simulink model "AMCLIB_BemfObsrvDQ_BAM"  (Simulink 9.3)
settings: Solver=VariableStepAuto  StartTime=0.0  StopTime=10.0  RelTol=1e-3
settings Model: Creator=nxa18952  LastModifiedBy=nxa18952
settings DataIOCC: SaveFormat=Dataset  SignalLoggingSaveFormat=Dataset  ReturnWorkspaceOutputs=on
settings OptimizationCC: LifeSpan=auto
settings DebuggingCC: UnderspecifiedInitializationDetection=Simplified  MergeDetectMultiDrivingBlocksExec=error  FcnCallInpInsideContextMsg=error  SFUnexpectedBacktrackingDiag=error  SFNoUnconditionalDefaultTransitionDiag=error  SFExecutionAtInitializationDiag=warning  ArithmeticOperatorsInVariantConditions=error
settings HardwareCC: ProdBitPerPointer=64  ProdBitPerSizeT=64  ProdBitPerPtrDiffT=64  ProdLargestAtomicFloat=Float  ProdIntDivRoundTo=Zero  ProdEndianess=LittleEndian  ProdWordSize=64  ProdHWDeviceType=Intel->x86-64 (Windows64)
settings ModelReferenceCC: PropagateSignalLabelsOutOfModel=on
settings SFSimCC: SimUseLocalCustomCode=on
settings RTWCC: RTWUseLocalCustomCode=on
settings CodeAppCC: StateflowObjectComments=off
settings GRTTargetCC: TargetLangStandard=C99 (ISO)  CombineOutputUpdateFcns=on  GRTInterface=off
settings ConfigComp: CovMetricSettings=dwe  CovHtmlReporting=off  CovSaveCumulativeToWorkspaceVar=off  CovSaveSingleToWorkspaceVar=off  CovExternalEMLEnable=on

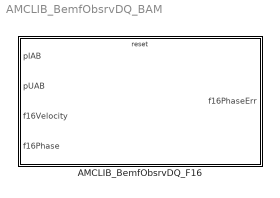
== system AMCLIB_BemfObsrvDQ_BAM ==
  AMCLIB_BemfObsrvDQ_F16 : Subsystem  TreatAsAtomicUnit=on  mask(AMCLIB_BemfObsrvDQ_F16){showStates=Hide (faster execution), resetStatesEnable=Pre-set according to the first set of inputs after reset, f16IGain=0, f16UGain=0, f16WIGain=0, f16EGain=0, s16Shift=0, f16CC1sc_D=0, f16CC2sc_D=0, f16UpperLimit_D=0, f16LowerLimit_D=0, f16CC1sc_Q=0, f16CC2sc_Q=0, f16UpperLimit_Q=0, f16LowerLimit_Q=0, u16NShift=0}
      mask prompts: showStates "Show internal states"; resetStatesEnable "Internal state after reset"; f16IGain "f16IGain (Scaled RL circuit constant)"; f16UGain "f16UGain (Scaled voltage cross-coupling constant)"; f16WIGain "f16WIGain (Scaled angular velocity cross-coupling constant)"; f16EGain "f16EGain (Scaled back-EMF cross-coupling constant)"; s16Shift "s16Shift (Scaling bitwise shift applied to all cross-coupling constants)"; f16CC1sc_D "f16CC1sc_D (CC1 coefficient of the D-axis PI controller)"; f16CC2sc_D "f16CC2sc_D (CC2 coefficient of the D-axis PI controller)"; f16UpperLimit_D "f16UpperLimit_D (Upper Limit of the D-axis PI controller)"; f16LowerLimit_D "f16LowerLimit_D (Lower Limit of the D-axis PI controller)"; f16CC1sc_Q "f16CC1sc_Q (CC1 coefficient of the Q-axis PI controller)"; f16CC2sc_Q "f16CC2sc_Q (CC2 coefficient of the Q-axis PI controller)"; f16UpperLimit_Q "f16UpperLimit_Q (Upper Limit of the Q-axis PI controller)"; f16LowerLimit_Q "f16LowerLimit_Q (Lower Limit of the Q-axis PI controller)"; u16NShift "u16NShift (Scaling bitwise shift applied to the controller coefficients)"
      mask help: PMSM back-EMF observer DQ in 16-bit fixed-point fractional implementation. This block supports re-initialization of the internal state during simulation. If the block is reset, the observer will align with the motor's position and speed measured in the next time step. This allows seamless on-the-fly transition to the closed-loop control. Refer to the AMMCLIB User's Guide for further details.
      mask init:
      | if ~evalin('base','exist(''tS8'',''var'')')
      |   if (2 ~= exist('SWLIBS_Typedefs.mat','file'))
      |       error('File SWLIBS_Typedefs.mat is not on the Matlab path. Please add the AMMCLIB "bam" folder in the Matlab Search Path.');
      |   else
      |       evalin('base', 'load(''SWLIBS_Typedefs.mat'')');
      |   end
      | end
      | if showStates == 1
      |     % hidden state variables
      |     if strcmp(get_param([gcb '/f16IGain'], 'BlockType'), 'Inport')
      |         posblk = get_param(gcb, 'Position');
      | 
      |         pos = get_param(    [gcb, '/f16IGain'], 'Position');
      |         orient = get_param( [gcb, '/f16IGain'], 'Orientation');
      |         delete_block(       [gcb, '/f16IGain']);
      |         add_block('built-in/Ground', [gcb, '/f16IGain'], 'Position', pos, 'Orientation', orient);
      | 
      |         pos = get_param(    [gcb, '/f16UGain'], 'Position');
      |         orient = get_param( [gcb, '/f16UGain'], 'Orientation');
      |         delete_block(       [gcb, '/f16UGain']);
      |         add_block('built-in/Ground', [gcb, '/f16UGain'], 'Position', pos, 'Orientation', orient);
      | 
      |         pos = get_param(    [gcb, '/f16WIGain'], 'Position');
      |         orient = get_param( [gcb, '/f16WIGain'], 'Orientation');
      |         delete_block(       [gcb, '/f16WIGain']);
      |         add_block('built-in/Ground', [gcb, '/f16WIGain'], 'Position', pos, 'Orientation', orient);
      | 
      |         pos = get_param(    [gcb, '/f16EGain'], 'Position');
      |         orient = get_param( [gcb, '/f16EGain'], 'Orientation');
      |         delete_block(       [gcb, '/f16EGain']);
      |         add_block('built-in/Ground', [gcb, '/f16EGain'], 'Position', pos, 'Orientation', orient);
      | 
      |         pos = get_param(    [gcb, '/s16Shift'], 'Position');
      |         orient = get_param( [gcb, '/s16Shift'], 'Orientation');
      |         delete_block(       [gcb, '/s16Shift']);
      |         add_block('built-in/Ground', [gcb, '/s16Shift'], 'Position', pos, 'Orientation', orient);
      | 
      |         pos = get_param(    [gcb, '/f16CC1sc_D'], 'Position');
      |         orient = get_param( [gcb, '/f16CC1sc_D'], 'Orientation');
      |         delete_block(       [gcb, '/f16CC1sc_D']);
      |         add_block('built-in/Ground', [gcb, '/f16CC1sc_D'], 'Position', pos, 'Orientation', orient);
      | 
      |         pos = get_param(    [gcb, '/f16CC2sc_D'], 'Position');
      |         orient = get_param( [gcb, '/f16CC2sc_D'], 'Orientation');
      |         delete_block(       [gcb, '/f16CC2sc_D']);
      |         add_block('built-in/Ground', [gcb, '/f16CC2sc_D'], 'Position', pos, 'Orientation', orient);
      | 
      |         pos = get_param(    [gcb, '/f16UpperLimit_D'], 'Position');
      |         orient = get_param( [gcb, '/f16UpperLimit_D'], 'Orientation');
      |         delete_block(       [gcb, '/f16UpperLimit_D']);
      |         add_block('built-in/Ground', [gcb, '/f16UpperLimit_D'], 'Position', pos, 'Orientation', orient);
      | 
      |         pos = get_param(    [gcb, '/f16LowerLimit_D'], 'Position');
      |         orient = get_param( [gcb, '/f16LowerLimit_D'], 'Orientation');
      |         delete_block(       [gcb, '/f16LowerLimit_D']);
      |         add_block('built-in/Ground', [gcb, '/f16LowerLimit_D'], 'Position', pos, 'Orientation', orient);
      | 
      |         pos = get_param(    [gcb, '/f16CC1sc_Q'], 'Position');
      |         orient = get_param( [gcb, '/f16CC1sc_Q'], 'Orientation');
      |         delete_block(       [gcb, '/f16CC1sc_Q']);
      |         add_block('built-in/Ground', [gcb, '/f16CC1sc_Q'], 'Position', pos, 'Orientation', orient);
      | 
      |         pos = get_param(    [gcb, '/f16CC2sc_Q'], 'Position');
      |         orient = get_param( [gcb, '/f16CC2sc_Q'], 'Orientation');
      |         delete_block(       [gcb, '/f16CC2sc_Q']);
      |         add_block('built-in/Ground', [gcb, '/f16CC2sc_Q'], 'Position', pos, 'Orientation', orient);
      | 
      |         pos = get_param(    [gcb, '/f16UpperLimit_Q'], 'Position');
      |         orient = get_param( [gcb, '/f16UpperLimit_Q'], 'Orientation');
      |         delete_block(       [gcb, '/f16UpperLimit_Q']);
      |         add_block('built-in/Ground', [gcb, '/f16UpperLimit_Q'], 'Position', pos, 'Orientation', orient);
      | 
      |         pos = get_param(    [gcb, '/f16LowerLimit_Q'], 'Position');
      |         orient = get_param( [gcb, '/f16LowerLimit_Q'], 'Orientation');
      |         delete_block(       [gcb, '/f16LowerLimit_Q']);
      |         add_block('built-in/Ground', [gcb, '/f16LowerLimit_Q'], 'Position', pos, 'Orientation', orient);
      | 
      |         pos = get_param(    [gcb, '/u16NShift'], 'Position');
      |         orient = get_param( [gcb, '/u16NShift'], 'Orientation');
      |         delete_block(       [gcb, '/u16NShift']);
      |         add_block('built-in/Ground', [gcb, '/u16NShift'], 'Position', pos, 'Orientation', orient);
      | 
      |         pos = get_param(    [gcb, '/f32Acc_D'], 'Position');
      |         orient = get_param( [gcb, '/f32Acc_D'], 'Orientation');
      |         delete_block(       [gcb, '/f32Acc_D']);
      |         add_block('built-in/Ground', [gcb, '/f32Acc_D'], 'Position', pos, 'Orientation', orient);
      | 
      |         pos = get_param(    [gcb, '/f16InErrK1_D'], 'Position');
      |         orient = get_param( [gcb, '/f16InErrK1_D'], 'Orientation');
      |         delete_block(       [gcb, '/f16InErrK1_D']);
      |         add_block('built-in/Ground', [gcb, '/f16InErrK1_D'], 'Position', pos, 'Orientation', orient);
      | 
      |         pos = get_param(    [gcb, '/f32Acc_Q'], 'Position');
      |         orient = get_param( [gcb, '/f32Acc_Q'], 'Orientation');
      |         delete_block(       [gcb, '/f32Acc_Q']);
      |         add_block('built-in/Ground', [gcb, '/f32Acc_Q'], 'Position', pos, 'Orientation', orient);
      | 
      |         pos = get_param(    [gcb, '/f16InErrK1_Q'], 'Position');
      |         orient = get_param( [gcb, '/f16InErrK1_Q'], 'Orientation');
      |         delete_block(       [gcb, '/f16InErrK1_Q']);
      |         add_block('built-in/Ground', [gcb, '/f16InErrK1_Q'], 'Position', pos, 'Orientation', orient);
      | 
      |         pos = get_param(    [gcb, '/f32IObsrvIn_1L_D'], 'Position');
      |         orient = get_param( [gcb, '/f32IObsrvIn_1L_D'], 'Orientation');
      |         delete_block(       [gcb, '/f32IObsrvIn_1L_D']);
      |         add_block('built-in/Ground', [gcb, '/f32IObsrvIn_1L_D'], 'Position', pos, 'Orientation', orient);
      | 
      |         pos = get_param(    [gcb, '/f16IObsrvIn_1H_D'], 'Position');
      |         orient = get_param( [gcb, '/f16IObsrvIn_1H_D'], 'Orientation');
      |         delete_block(       [gcb, '/f16IObsrvIn_1H_D']);
      |         add_block('built-in/Ground', [gcb, '/f16IObsrvIn_1H_D'], 'Position', pos, 'Orientation', orient);
      | 
      |         pos = get_param(    [gcb, '/f32IObsrvIn_1L_Q'], 'Position');
      |         orient = get_param( [gcb, '/f32IObsrvIn_1L_Q'], 'Orientation');
      |         delete_block(       [gcb, '/f32IObsrvIn_1L_Q']);
      |         add_block('built-in/Ground', [gcb, '/f32IObsrvIn_1L_Q'], 'Position', pos, 'Orientation', orient);
      | 
      |         pos = get_param(    [gcb, '/f16IObsrvIn_1H_Q'], 'Position');
      |         orient = get_param( [gcb, '/f16IObsrvIn_1H_Q'], 'Orientation');
      |         delete_block(       [gcb, '/f16IObsrvIn_1H_Q']);
      |         add_block('built-in/Ground', [gcb, '/f16IObsrvIn_1H_Q'], 'Position', pos, 'Orientation', orient);
      | 
      |         pos = get_param(    [gcb, '/f32IObsrv_D'], 'Position');
      |         orient = get_param( [gcb, '/f32IObsrv_D'], 'Orientation');
      |         delete_block(       [gcb, '/f32IObsrv_D']);
      |         add_block('built-in/Ground', [gcb, '/f32IObsrv_D'], 'Position', pos, 'Orientation', orient);
      | 
      |         pos = get_param(    [gcb, '/f32IObsrv_Q'], 'Position');
      |         orient = get_param( [gcb, '/f32IObsrv_Q'], 'Orientation');
      |         delete_block(       [gcb, '/f32IObsrv_Q']);
      |         add_block('built-in/Ground', [gcb, '/f32IObsrv_Q'], 'Position', pos, 'Orientation', orient);
      | 
      | 
      |         pos = get_param(    [gcb '/f16EObsrv_D_Out'], 'Position');
      |         orient = get_param( [gcb '/f16EObsrv_D_Out'], 'Orientation');
      |         delete_block(       [gcb '/f16EObsrv_D_Out']);
      |         add_block('built-in/Terminator', [gcb '/f16EObsrv_D_Out'], 'Position', pos, 'Orientation', orient);
      | 
      |         pos = get_param(    [gcb '/f16EObsrv_Q_Out'], 'Position');
      |         orient = get_param( [gcb '/f16EObsrv_Q_Out'], 'Orientation');
      |         delete_block(       [gcb '/f16EObsrv_Q_Out']);
      |         add_block('built-in/Terminator', [gcb '/f16EObsrv_Q_Out'], 'Position', pos, 'Orientation', orient);
      | 
      |         pos = get_param(    [gcb '/f32Acc_D_Out'], 'Position');
      |         orient = get_param( [gcb '/f32Acc_D_Out'], 'Orientation');
      |         delete_block(       [gcb '/f32Acc_D_Out']);
      |         add_block('built-in/Terminator', [gcb '/f32Acc_D_Out'], 'Position', pos, 'Orientation', orient);
      | 
      |         pos = get_param(    [gcb '/f16InErrK1_D_Out'], 'Position');
      |         orient = get_param( [gcb '/f16InErrK1_D_Out'], 'Orientation');
      |         delete_block(       [gcb '/f16InErrK1_D_Out']);
      |         add_block('built-in/Terminator', [gcb '/f16InErrK1_D_Out'], 'Position', pos, 'Orientation', orient);
      | 
      |         pos = get_param(    [gcb '/f32Acc_Q_Out'], 'Position');
      |         orient = get_param( [gcb '/f32Acc_Q_Out'], 'Orientation');
      |         delete_block(       [gcb '/f32Acc_Q_Out']);
      |         add_block('built-in/Terminator', [gcb '/f32Acc_Q_Out'], 'Position', pos, 'Orientation', orient);
      | 
      |         pos = get_param(    [gcb '/f16InErrK1_Q_Out'], 'Position');
      |         orient = get_param( [gcb '/f16InErrK1_Q_Out'], 'Orientation');
      |         delete_block(       [gcb '/f16InErrK1_Q_Out']);
      |         add_block('built-in/Terminator', [gcb '/f16InErrK1_Q_Out'], 'Position', pos, 'Orientation', orient);
      | 
      |         pos = get_param(    [gcb '/f32IObsrvIn_1L_D_Out'], 'Position');
      |         orient = get_param( [gcb '/f32IObsrvIn_1L_D_Out'], 'Orientation');
      |         delete_block(       [gcb '/f32IObsrvIn_1L_D_Out']);
      |         add_block('built-in/Terminator', [gcb '/f32IObsrvIn_1L_D_Out'], 'Position', pos, 'Orientation', orient);
      | 
      |         pos = get_param(    [gcb '/f16IObsrvIn_1H_D_Out'], 'Position');
      |         orient = get_param( [gcb '/f16IObsrvIn_1H_D_Out'], 'Orientation');
      |         delete_block(       [gcb '/f16IObsrvIn_1H_D_Out']);
      |         add_block('built-in/Terminator', [gcb '/f16IObsrvIn_1H_D_Out'], 'Position', pos, 'Orientation', orient);
      | 
      |         pos = get_param(    [gcb '/f32IObsrvIn_1L_Q_Out'], 'Position');
      |         orient = get_param( [gcb '/f32IObsrvIn_1L_Q_Out'], 'Orientation');
      |         delete_block(       [gcb '/f32IObsrvIn_1L_Q_Out']);
      |         add_block('built-in/Terminator', [gcb '/f32IObsrvIn_1L_Q_Out'], 'Position', pos, 'Orientation', orient);
      | 
      |         pos = get_param(    [gcb '/f16IObsrvIn_1H_Q_Out'], 'Position');
      |         orient = get_param( [gcb '/f16IObsrvIn_1H_Q_Out'], 'Orientation');
      |         delete_block(       [gcb '/f16IObsrvIn_1H_Q_Out']);
      |         add_block('built-in/Terminator', [gcb '/f16IObsrvIn_1H_Q_Out'], 'Position', pos, 'Orientation', orient);
      | 
      |         pos = get_param(    [gcb '/f32IObsrv_D_Out'], 'Position');
      |         orient = get_param( [gcb '/f32IObsrv_D_Out'], 'Orientation');
      |         delete_block(       [gcb '/f32IObsrv_D_Out']);
      |         add_block('built-in/Terminator', [gcb '/f32IObsrv_D_Out'], 'Position', pos, 'Orientation', orient);
      | 
      |         pos = get_param(    [gcb '/f32IObsrv_Q_Out'], 'Position');
      |         orient = get_param( [gcb '/f32IObsrv_Q_Out'], 'Orientation');
      |         delete_block(       [gcb '/f32IObsrv_Q_Out']);
      |         add_block('built-in/Terminator', [gcb '/f32IObsrv_Q_Out'], 'Position', pos, 'Orientation', orient);
      | 
      | 
      |         set_param([gcb '/pIAB'], 'Port', '1');
      |         set_param([gcb '/pUAB'], 'Port', '2');
      |         set_param([gcb '/f16Velocity'], 'Port', '3');
      |         set_param([gcb '/f16Phase'], 'Port', '4');
      | 
      |         set_param([gcb '/f16PhaseErr'], 'Port', '1');
      | 
      |         set_param(gcb,'MaskEnables',{'on','on','on','on','on','on','on','on','on','on','on','on','on','on','on','on'});
      | 
      |         if (posblk(4) - posblk(2)) > 125
      |           height = 125;
      |           set_param(gcb,'Position',[posblk(1), posblk(2), posblk(3), posblk(2)+height])
      |         end
      |     end
      | else
      |     % shown state variables
      |     if strcmp(get_param([gcb '/f16IGain'], 'BlockType'), 'Ground')
      |         posblk = get_param(gcb, 'Position');
      | 
      |         pos = get_param(    [gcb, '/f16IGain'], 'Position');
      |         orient = get_param( [gcb, '/f16IGain'], 'Orientation');
      |         delete_block(       [gcb, '/f16IGain']);
      |         add_block('built-in/Inport', [gcb, '/f16IGain'], 'Position', pos, 'Orientation', orient, 'OutDataTypeStr', 'int16');
      | 
      |         pos = get_param(    [gcb, '/f16UGain'], 'Position');
      |         orient = get_param( [gcb, '/f16UGain'], 'Orientation');
      |         delete_block(       [gcb, '/f16UGain']);
      |         add_block('built-in/Inport', [gcb, '/f16UGain'], 'Position', pos, 'Orientation', orient, 'OutDataTypeStr', 'int16');
      | 
      |         pos = get_param(    [gcb, '/f16WIGain'], 'Position');
      |         orient = get_param( [gcb, '/f16WIGain'], 'Orientation');
      |         delete_block(       [gcb, '/f16WIGain']);
      |         add_block('built-in/Inport', [gcb, '/f16WIGain'], 'Position', pos, 'Orientation', orient, 'OutDataTypeStr', 'int16');
      | 
      |         pos = get_param(    [gcb, '/f16EGain'], 'Position');
      |         orient = get_param( [gcb, '/f16EGain'], 'Orientation');
      |         delete_block(       [gcb, '/f16EGain']);
      |         add_block('built-in/Inport', [gcb, '/f16EGain'], 'Position', pos, 'Orientation', orient, 'OutDataTypeStr', 'int16');
      | 
      |         pos = get_param(    [gcb, '/s16Shift'], 'Position');
      |         orient = get_param( [gcb, '/s16Shift'], 'Orientation');
      |         delete_block(       [gcb, '/s16Shift']);
      |         add_block('built-in/Inport', [gcb, '/s16Shift'], 'Position', pos, 'Orientation', orient, 'OutDataTypeStr', 'int16');
      | 
      |         pos = get_param(    [gcb, '/f16CC1sc_D'], 'Position');
      |         orient = get_param( [gcb, '/f16CC1sc_D'], 'Orientation');
      |         delete_block(       [gcb, '/f16CC1sc_D']);
      |         add_block('built-in/Inport', [gcb, '/f16CC1sc_D'], 'Position', pos, 'Orientation', orient, 'OutDataTypeStr', 'int16');
      | 
      |         pos = get_param(    [gcb, '/f16CC2sc_D'], 'Position');
      |         orient = get_param( [gcb, '/f16CC2sc_D'], 'Orientation');
      |         delete_block(       [gcb, '/f16CC2sc_D']);
      |         add_block('built-in/Inport', [gcb, '/f16CC2sc_D'], 'Position', pos, 'Orientation', orient, 'OutDataTypeStr', 'int16');
      | 
      |         pos = get_param(    [gcb, '/f16UpperLimit_D'], 'Position');
      |         orient = get_param( [gcb, '/f16UpperLimit_D'], 'Orientation');
      |         delete_block(       [gcb, '/f16UpperLimit_D']);
      |         add_block('built-in/Inport', [gcb, '/f16UpperLimit_D'], 'Position', pos, 'Orientation', orient, 'OutDataTypeStr', 'int16');
      | 
      |         pos = get_param(    [gcb, '/f16LowerLimit_D'], 'Position');
      |         orient = get_param( [gcb, '/f16LowerLimit_D'], 'Orientation');
      |         delete_block(       [gcb, '/f16LowerLimit_D']);
      |         add_block('built-in/Inport', [gcb, '/f16LowerLimit_D'], 'Position', pos, 'Orientation', orient, 'OutDataTypeStr', 'int16');
      | 
      |         pos = get_param(    [gcb, '/f16CC1sc_Q'], 'Position');
      |         orient = get_param( [gcb, '/f16CC1sc_Q'], 'Orientation');
      |         delete_block(       [gcb, '/f16CC1sc_Q']);
      |         add_block('built-in/Inport', [gcb, '/f16CC1sc_Q'], 'Position', pos, 'Orientation', orient, 'OutDataTypeStr', 'int16');
      | 
      |         pos = get_param(    [gcb, '/f16CC2sc_Q'], 'Position');
      |         orient = get_param( [gcb, '/f16CC2sc_Q'], 'Orientation');
      |         delete_block(       [gcb, '/f16CC2sc_Q']);
      |         add_block('built-in/Inport', [gcb, '/f16CC2sc_Q'], 'Position', pos, 'Orientation', orient, 'OutDataTypeStr', 'int16');
      | 
      |         pos = get_param(    [gcb, '/f16UpperLimit_Q'], 'Position');
      |         orient = get_param( [gcb, '/f16UpperLimit_Q'], 'Orientation');
      |         delete_block(       [gcb, '/f16UpperLimit_Q']);
      |         add_block('built-in/Inport', [gcb, '/f16UpperLimit_Q'], 'Position', pos, 'Orientation', orient, 'OutDataTypeStr', 'int16');
      | 
      |         pos = get_param(    [gcb, '/f16LowerLimit_Q'], 'Position');
      |         orient = get_param( [gcb, '/f16LowerLimit_Q'], 'Orientation');
      |         delete_block(       [gcb, '/f16LowerLimit_Q']);
      |         add_block('built-in/Inport', [gcb, '/f16LowerLimit_Q'], 'Position', pos, 'Orientation', orient, 'OutDataTypeStr', 'int16');
      | 
      |         pos = get_param(    [gcb, '/u16NShift'], 'Position');
      |         orient = get_param( [gcb, '/u16NShift'], 'Orientation');
      |         delete_block(       [gcb, '/u16NShift']);
      |         add_block('built-in/Inport', [gcb, '/u16NShift'], 'Position', pos, 'Orientation', orient, 'OutDataTypeStr', 'uint16');
      | 
      |         pos = get_param(    [gcb, '/f32Acc_D'], 'Position');
      |         orient = get_param( [gcb, '/f32Acc_D'], 'Orientation');
      |         delete_block(       [gcb, '/f32Acc_D']);
      |         add_block('built-in/Inport', [gcb, '/f32Acc_D'], 'Position', pos, 'Orientation', orient, 'OutDataTypeStr', 'int32');
      | 
      |         pos = get_param(    [gcb, '/f16InErrK1_D'], 'Position');
      |         orient = get_param( [gcb, '/f16InErrK1_D'], 'Orientation');
      |         delete_block(       [gcb, '/f16InErrK1_D']);
      |         add_block('built-in/Inport', [gcb, '/f16InErrK1_D'], 'Position', pos, 'Orientation', orient, 'OutDataTypeStr', 'int16');
      | 
      |         pos = get_param(    [gcb, '/f32Acc_Q'], 'Position');
      |         orient = get_param( [gcb, '/f32Acc_Q'], 'Orientation');
      |         delete_block(       [gcb, '/f32Acc_Q']);
      |         add_block('built-in/Inport', [gcb, '/f32Acc_Q'], 'Position', pos, 'Orientation', orient, 'OutDataTypeStr', 'int32');
      | 
      |         pos = get_param(    [gcb, '/f16InErrK1_Q'], 'Position');
      |         orient = get_param( [gcb, '/f16InErrK1_Q'], 'Orientation');
      |         delete_block(       [gcb, '/f16InErrK1_Q']);
      |         add_block('built-in/Inport', [gcb, '/f16InErrK1_Q'], 'Position', pos, 'Orientation', orient, 'OutDataTypeStr', 'int16');
      | 
      |         pos = get_param(    [gcb, '/f32IObsrvIn_1L_D'], 'Position');
      |         orient = get_param( [gcb, '/f32IObsrvIn_1L_D'], 'Orientation');
      |         delete_block(       [gcb, '/f32IObsrvIn_1L_D']);
      |         add_block('built-in/Inport', [gcb, '/f32IObsrvIn_1L_D'], 'Position', pos, 'Orientation', orient, 'OutDataTypeStr', 'int32');
      | 
      |         pos = get_param(    [gcb, '/f16IObsrvIn_1H_D'], 'Position');
      |         orient = get_param( [gcb, '/f16IObsrvIn_1H_D'], 'Orientation');
      |         delete_block(       [gcb, '/f16IObsrvIn_1H_D']);
      |         add_block('built-in/Inport', [gcb, '/f16IObsrvIn_1H_D'], 'Position', pos, 'Orientation', orient, 'OutDataTypeStr', 'int16');
      | 
      |         pos = get_param(    [gcb, '/f32IObsrvIn_1L_Q'], 'Position');
      |         orient = get_param( [gcb, '/f32IObsrvIn_1L_Q'], 'Orientation');
      |         delete_block(       [gcb, '/f32IObsrvIn_1L_Q']);
      |         add_block('built-in/Inport', [gcb, '/f32IObsrvIn_1L_Q'], 'Position', pos, 'Orientation', orient, 'OutDataTypeStr', 'int32');
      | 
      |         pos = get_param(    [gcb, '/f16IObsrvIn_1H_Q'], 'Position');
      |         orient = get_param( [gcb, '/f16IObsrvIn_1H_Q'], 'Orientation');
      |         delete_block(       [gcb, '/f16IObsrvIn_1H_Q']);
      |         add_block('built-in/Inport', [gcb, '/f16IObsrvIn_1H_Q'], 'Position', pos, 'Orientation', orient, 'OutDataTypeStr', 'int16');
      | 
      |         pos = get_param(    [gcb, '/f32IObsrv_D'], 'Position');
      |         orient = get_param( [gcb, '/f32IObsrv_D'], 'Orientation');
      |         delete_block(       [gcb, '/f32IObsrv_D']);
      |         add_block('built-in/Inport', [gcb, '/f32IObsrv_D'], 'Position', pos, 'Orientation', orient, 'OutDataTypeStr', 'int32');
      | 
      |         pos = get_param(    [gcb, '/f32IObsrv_Q'], 'Position');
      |         orient = get_param( [gcb, '/f32IObsrv_Q'], 'Orientation');
      |         delete_block(       [gcb, '/f32IObsrv_Q']);
      |         add_block('built-in/Inport', [gcb, '/f32IObsrv_Q'], 'Position', pos, 'Orientation', orient, 'OutDataTypeStr', 'int32');
      | 
      | 
      |         pos = get_param(    [gcb '/f16EObsrv_D_Out'], 'Position');
      |         orient = get_param( [gcb '/f16EObsrv_D_Out'], 'Orientation');
      |         delete_block(       [gcb '/f16EObsrv_D_Out']);
      |         add_block('built-in/Outport', [gcb '/f16EObsrv_D_Out'], 'Position', pos, 'Orientation', orient);
      | 
      |         pos = get_param(    [gcb '/f16EObsrv_Q_Out'], 'Position');
      |         orient = get_param( [gcb '/f16EObsrv_Q_Out'], 'Orientation');
      |         delete_block(       [gcb '/f16EObsrv_Q_Out']);
      |         add_block('built-in/Outport', [gcb '/f16EObsrv_Q_Out'], 'Position', pos, 'Orientation', orient);
      | 
      |         pos = get_param(    [gcb '/f32Acc_D_Out'], 'Position');
      |         orient = get_param( [gcb '/f32Acc_D_Out'], 'Orientation');
      |         delete_block(       [gcb '/f32Acc_D_Out']);
      |         add_block('built-in/Outport', [gcb '/f32Acc_D_Out'], 'Position', pos, 'Orientation', orient);
      | 
      |         pos = get_param(    [gcb '/f16InErrK1_D_Out'], 'Position');
      |         orient = get_param( [gcb '/f16InErrK1_D_Out'], 'Orientation');
      |         delete_block(       [gcb '/f16InErrK1_D_Out']);
      |         add_block('built-in/Outport', [gcb '/f16InErrK1_D_Out'], 'Position', pos, 'Orientation', orient);
      | 
      |         pos = get_param(    [gcb '/f32Acc_Q_Out'], 'Position');
      |         orient = get_param( [gcb '/f32Acc_Q_Out'], 'Orientation');
      |         delete_block(       [gcb '/f32Acc_Q_Out']);
      |         add_block('built-in/Outport', [gcb '/f32Acc_Q_Out'], 'Position', pos, 'Orientation', orient);
      | 
      |         pos = get_param(    [gcb '/f16InErrK1_Q_Out'], 'Position');
      |         orient = get_param( [gcb '/f16InErrK1_Q_Out'], 'Orientation');
      |         delete_block(       [gcb '/f16InErrK1_Q_Out']);
      |         add_block('built-in/Outport', [gcb '/f16InErrK1_Q_Out'], 'Position', pos, 'Orientation', orient);
      | 
      |         pos = get_param(    [gcb '/f32IObsrvIn_1L_D_Out'], 'Position');
      |         orient = get_param( [gcb '/f32IObsrvIn_1L_D_Out'], 'Orientation');
      |         delete_block(       [gcb '/f32IObsrvIn_1L_D_Out']);
      |         add_block('built-in/Outport', [gcb '/f32IObsrvIn_1L_D_Out'], 'Position', pos, 'Orientation', orient);
      | 
      |         pos = get_param(    [gcb '/f16IObsrvIn_1H_D_Out'], 'Position');
      |         orient = get_param( [gcb '/f16IObsrvIn_1H_D_Out'], 'Orientation');
      |         delete_block(       [gcb '/f16IObsrvIn_1H_D_Out']);
      |         add_block('built-in/Outport', [gcb '/f16IObsrvIn_1H_D_Out'], 'Position', pos, 'Orientation', orient);
      | 
      |         pos = get_param(    [gcb '/f32IObsrvIn_1L_Q_Out'], 'Position');
      |         orient = get_param( [gcb '/f32IObsrvIn_1L_Q_Out'], 'Orientation');
      |         delete_block(       [gcb '/f32IObsrvIn_1L_Q_Out']);
      |         add_block('built-in/Outport', [gcb '/f32IObsrvIn_1L_Q_Out'], 'Position', pos, 'Orientation', orient);
      | 
      |         pos = get_param(    [gcb '/f16IObsrvIn_1H_Q_Out'], 'Position');
      |         orient = get_param( [gcb '/f16IObsrvIn_1H_Q_Out'], 'Orientation');
      |         delete_block(       [gcb '/f16IObsrvIn_1H_Q_Out']);
      |         add_block('built-in/Outport', [gcb '/f16IObsrvIn_1H_Q_Out'], 'Position', pos, 'Orientation', orient);
      | 
      |         pos = get_param(    [gcb '/f32IObsrv_D_Out'], 'Position');
      |         orient = get_param( [gcb '/f32IObsrv_D_Out'], 'Orientation');
      |         delete_block(       [gcb '/f32IObsrv_D_Out']);
      |         add_block('built-in/Outport', [gcb '/f32IObsrv_D_Out'], 'Position', pos, 'Orientation', orient);
      | 
      |         pos = get_param(    [gcb '/f32IObsrv_Q_Out'], 'Position');
      |         orient = get_param( [gcb '/f32IObsrv_Q_Out'], 'Orientation');
      |         delete_block(       [gcb '/f32IObsrv_Q_Out']);
      |         add_block('built-in/Outport', [gcb '/f32IObsrv_Q_Out'], 'Position', pos, 'Orientation', orient);
      | 
      | 
      |         set_param([gcb '/pIAB'], 'Port', '1');
      |         set_param([gcb '/pUAB'], 'Port', '2');
      |         set_param([gcb '/f16Velocity'], 'Port', '3');
      |         set_param([gcb '/f16Phase'], 'Port', '4');
      |         set_param([gcb '/f16IGain'], 'Port', '5');
      |         set_param([gcb '/f16UGain'], 'Port', '6');
      |         set_param([gcb '/f16WIGain'], 'Port', '7');
      |         set_param([gcb '/f16EGain'], 'Port', '8');
      |         set_param([gcb '/s16Shift'], 'Port', '9');
      |         set_param([gcb '/f16CC1sc_D'], 'Port', '10');
      |         set_param([gcb '/f16CC2sc_D'], 'Port', '11');
      |         set_param([gcb '/f16UpperLimit_D'], 'Port', '12');
      |         set_param([gcb '/f16LowerLimit_D'], 'Port', '13');
      |         set_param([gcb '/f16CC1sc_Q'], 'Port', '14');
      |         set_param([gcb '/f16CC2sc_Q'], 'Port', '15');
      |         set_param([gcb '/f16UpperLimit_Q'], 'Port', '16');
      |         set_param([gcb '/f16LowerLimit_Q'], 'Port', '17');
      |         set_param([gcb '/u16NShift'], 'Port', '18');
      |         set_param([gcb '/f32Acc_D'], 'Port', '19');
      |         set_param([gcb '/f16InErrK1_D'], 'Port', '20');
      |         set_param([gcb '/f32Acc_Q'], 'Port', '21');
      |         set_param([gcb '/f16InErrK1_Q'], 'Port', '22');
      |         set_param([gcb '/f32IObsrvIn_1L_D'], 'Port', '23');
      |         set_param([gcb '/f16IObsrvIn_1H_D'], 'Port', '24');
      |         set_param([gcb '/f32IObsrvIn_1L_Q'], 'Port', '25');
      |         set_param([gcb '/f16IObsrvIn_1H_Q'], 'Port', '26');
      |         set_param([gcb '/f32IObsrv_D'], 'Port', '27');
      |         set_param([gcb '/f32IObsrv_Q'], 'Port', '28');
      | 
      |         set_param([gcb '/f16PhaseErr'], 'Port', '1');
      |         set_param([gcb '/f16EObsrv_D_Out'], 'Port', '2');
      |         set_param([gcb '/f16EObsrv_Q_Out'], 'Port', '3');
      |         set_param([gcb '/f32Acc_D_Out'], 'Port', '4');
      |         set_param([gcb '/f16InErrK1_D_Out'], 'Port', '5');
      |         set_param([gcb '/f32Acc_Q_Out'], 'Port', '6');
      |         set_param([gcb '/f16InErrK1_Q_Out'], 'Port', '7');
      |         set_param([gcb '/f32IObsrvIn_1L_D_Out'], 'Port', '8');
      |         set_param([gcb '/f16IObsrvIn_1H_D_Out'], 'Port', '9');
      |         set_param([gcb '/f32IObsrvIn_1L_Q_Out'], 'Port', '10');
      |         set_param([gcb '/f16IObsrvIn_1H_Q_Out'], 'Port', '11');
      |         set_param([gcb '/f32IObsrv_D_Out'], 'Port', '12');
      |         set_param([gcb '/f32IObsrv_Q_Out'], 'Port', '13');
      | 
      |         set_param(gcb,'MaskEnables',{'on','on','off','off','off','off','off','off','off','off','off','off','off','off','off','off'});
      | 
      |         if (posblk(4) - posblk(2)) < 725
      |           height = 725;
      |           set_param(gcb,'Position',[posblk(1), posblk(2), posblk(3), posblk(2)+height])
      |         end
      |     end
      | end
      settings: RTWSystemCode=Inline
      mask TypeOptions showStates: Hide (faster execution) | Show (allows debugging; connect feedback loops manually)
      mask Callback showStates:
      | maskStr = get_param(gcb,'showStates');
      | if strcmp(maskStr,'Hide (faster execution)'),
      |     set_param(gcb,'MaskEnables',{'on','on','on','on','on','on','on','on','on','on','on','on','on','on','on','on'});
      | else
      |     set_param(gcb,'MaskEnables',{'on','on','off','off','off','off','off','off','off','off','off','off','off','off','off','off'});
      | end
      mask TypeOptions resetStatesEnable: Pre-set according to the first set of inputs after reset | Clear to zero
      mask Display:
      | color('black');
      | pos = get_param(gcb, 'Position');
      | width = pos(3) - pos(1);
      | height = pos(4) - pos(2);
      | tX=width/2;
      | tY=height - 25;
      | color('black');
      | text(tX,tY, 'AMCLIB_BemfObsrvDQ_F16', 'horizontalAlignment', 'center');
      | if showStates == 2
      |   color('red');
      |   text(tX,tY - 20, ['debugging mode' char(13) char(10) '(limited performance)'], 'horizontalAlignment', 'center');
      | end

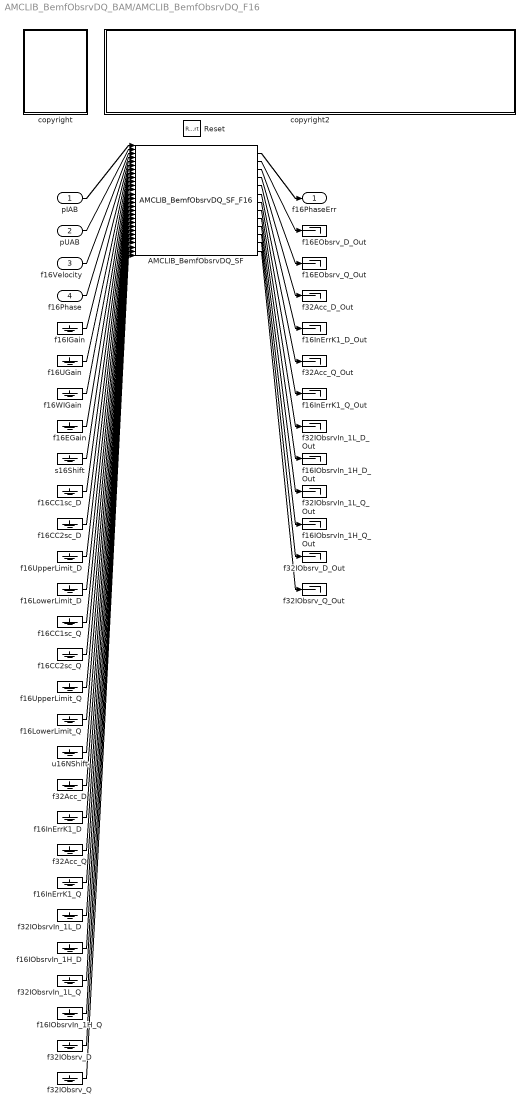
== system AMCLIB_BemfObsrvDQ_BAM/AMCLIB_BemfObsrvDQ_F16 ==
  pIAB : Inport  OutDataTypeStr=Bus: SWLIBS_2Syst_F16  BusOutputAsStruct=on
  pUAB : Inport  Port=2  OutDataTypeStr=Bus: SWLIBS_2Syst_F16  BusOutputAsStruct=on
  f16Velocity : Inport  Port=3  OutDataTypeStr=int16
  f16Phase : Inport  Port=4  OutDataTypeStr=int16
  Reset : ResetPort  DisableCoverage=on
  AMCLIB_BemfObsrvDQ_SF : S-Function  FunctionName=AMCLIB_BemfObsrvDQ_SF_F16  Parameters=showStates,resetStatesEnable,f16IGain,f16UGain,f16WIGain,f16EGain,s16Shift,f16CC1sc_D,f16CC2sc_D,f16UpperLimit_D,f16LowerLimit_D,f16CC1sc_Q,f16CC2sc_Q,f16UpperLimit_Q,f16LowerLimit_Q,u16NShift  SFunctionDeploymentMode=off  EnableBusSupport=off
  copyright : Subsystem
      mask Display: text(10,90,'FILE:');text(10,75,'DESRIPTION:');text(10,60,'COPYRIGHT:');text(10,45,'VERSION:');text(10,30,'DATE:')
  copyright2 : Subsystem
      mask Display: text(10,90,'AMCLIB_BemfObsrvDQ_BAM_F16.mdl');text(10,75,'PMSM back-EMF observer DQ.');text(10,60,'NXP 2020');text(10,45,'1.0');text(10,30,'28-Mar-2020');
  f16CC1sc_D : Ground
  f16CC1sc_Q : Ground
  f16CC2sc_D : Ground
  f16CC2sc_Q : Ground
  f16EGain : Ground
  f16EObsrv_D_Out : Terminator
  f16EObsrv_Q_Out : Terminator
  f16IGain : Ground
  f16IObsrvIn_1H_D : Ground
  f16IObsrvIn_1H_D_Out : Terminator
  f16IObsrvIn_1H_Q : Ground
  f16IObsrvIn_1H_Q_Out : Terminator
  f16InErrK1_D : Ground
  f16InErrK1_D_Out : Terminator
  f16InErrK1_Q : Ground
  f16InErrK1_Q_Out : Terminator
  f16LowerLimit_D : Ground
  f16LowerLimit_Q : Ground
  f16UGain : Ground
  f16UpperLimit_D : Ground
  f16UpperLimit_Q : Ground
  f16WIGain : Ground
  f32Acc_D : Ground
  f32Acc_D_Out : Terminator
  f32Acc_Q : Ground
  f32Acc_Q_Out : Terminator
  f32IObsrvIn_1L_D : Ground
  f32IObsrvIn_1L_D_Out : Terminator
  f32IObsrvIn_1L_Q : Ground
  f32IObsrvIn_1L_Q_Out : Terminator
  f32IObsrv_D : Ground
  f32IObsrv_D_Out : Terminator
  f32IObsrv_Q : Ground
  f32IObsrv_Q_Out : Terminator
  s16Shift : Ground
  u16NShift : Ground
  f16PhaseErr : Outport
  wires:
  pIAB/1 -> AMCLIB_BemfObsrvDQ_SF/1
  pUAB/1 -> AMCLIB_BemfObsrvDQ_SF/2
  f16Velocity/1 -> AMCLIB_BemfObsrvDQ_SF/3
  f16Phase/1 -> AMCLIB_BemfObsrvDQ_SF/4
  f16IGain/1 -> AMCLIB_BemfObsrvDQ_SF/5
  f16UGain/1 -> AMCLIB_BemfObsrvDQ_SF/6
  f16WIGain/1 -> AMCLIB_BemfObsrvDQ_SF/7
  f16EGain/1 -> AMCLIB_BemfObsrvDQ_SF/8
  s16Shift/1 -> AMCLIB_BemfObsrvDQ_SF/9
  f16CC1sc_D/1 -> AMCLIB_BemfObsrvDQ_SF/10
  f16CC2sc_D/1 -> AMCLIB_BemfObsrvDQ_SF/11
  f16UpperLimit_D/1 -> AMCLIB_BemfObsrvDQ_SF/12
  f16LowerLimit_D/1 -> AMCLIB_BemfObsrvDQ_SF/13
  f16CC1sc_Q/1 -> AMCLIB_BemfObsrvDQ_SF/14
  f16CC2sc_Q/1 -> AMCLIB_BemfObsrvDQ_SF/15
  f16UpperLimit_Q/1 -> AMCLIB_BemfObsrvDQ_SF/16
  f16LowerLimit_Q/1 -> AMCLIB_BemfObsrvDQ_SF/17
  u16NShift/1 -> AMCLIB_BemfObsrvDQ_SF/18
  f32Acc_D/1 -> AMCLIB_BemfObsrvDQ_SF/19
  f16InErrK1_D/1 -> AMCLIB_BemfObsrvDQ_SF/20
  f32Acc_Q/1 -> AMCLIB_BemfObsrvDQ_SF/21
  f16InErrK1_Q/1 -> AMCLIB_BemfObsrvDQ_SF/22
  f32IObsrvIn_1L_D/1 -> AMCLIB_BemfObsrvDQ_SF/23
  f16IObsrvIn_1H_D/1 -> AMCLIB_BemfObsrvDQ_SF/24
  f32IObsrvIn_1L_Q/1 -> AMCLIB_BemfObsrvDQ_SF/25
  f16IObsrvIn_1H_Q/1 -> AMCLIB_BemfObsrvDQ_SF/26
  f32IObsrv_D/1 -> AMCLIB_BemfObsrvDQ_SF/27
  f32IObsrv_Q/1 -> AMCLIB_BemfObsrvDQ_SF/28
  AMCLIB_BemfObsrvDQ_SF/1 -> f16PhaseErr/1
  AMCLIB_BemfObsrvDQ_SF/2 -> f16EObsrv_D_Out/1
  AMCLIB_BemfObsrvDQ_SF/3 -> f16EObsrv_Q_Out/1
  AMCLIB_BemfObsrvDQ_SF/4 -> f32Acc_D_Out/1
  AMCLIB_BemfObsrvDQ_SF/5 -> f16InErrK1_D_Out/1
  AMCLIB_BemfObsrvDQ_SF/6 -> f32Acc_Q_Out/1
  AMCLIB_BemfObsrvDQ_SF/7 -> f16InErrK1_Q_Out/1
  AMCLIB_BemfObsrvDQ_SF/8 -> f32IObsrvIn_1L_D_Out/1
  AMCLIB_BemfObsrvDQ_SF/9 -> f16IObsrvIn_1H_D_Out/1
  AMCLIB_BemfObsrvDQ_SF/10 -> f32IObsrvIn_1L_Q_Out/1
  AMCLIB_BemfObsrvDQ_SF/11 -> f16IObsrvIn_1H_Q_Out/1
  AMCLIB_BemfObsrvDQ_SF/12 -> f32IObsrv_D_Out/1
  AMCLIB_BemfObsrvDQ_SF/13 -> f32IObsrv_Q_Out/1

== system AMCLIB_BemfObsrvDQ_BAM/AMCLIB_BemfObsrvDQ_F16/copyright ==

== system AMCLIB_BemfObsrvDQ_BAM/AMCLIB_BemfObsrvDQ_F16/copyright2 ==
